simulink model "MODELO_SENOIDAL_SIMPLE"  (R2024b)
settings: Solver=VariableStepAuto  StartTime=0.0  StopTime=10.0  RelTol=1e-3
libraries: simulink x1
settings Model: Creator=RREYM  LastModifiedBy=RREYM

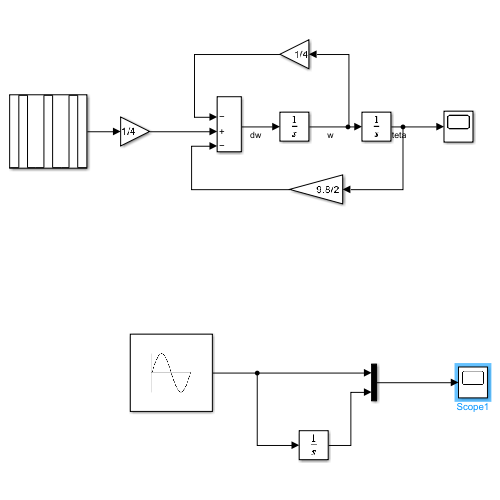
[thumbnail: Simulink's stored preview of the top-level diagram]
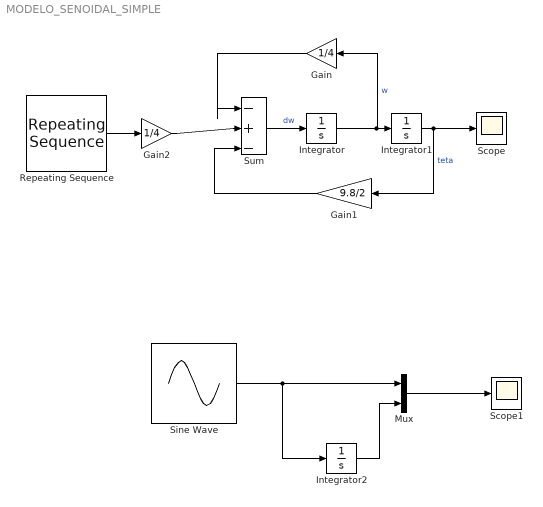
== system MODELO_SENOIDAL_SIMPLE ==
  Gain : Gain  Gain=1/4
  Gain1 : Gain  Gain=9.8/2
  Gain2 : Gain  Gain=1/4
  Integrator : Integrator
  Integrator1 : Integrator
  Integrator2 : Integrator
  Mux : Mux  Inputs=2
  Repeating Sequence : simulink/Sources/Repeating Sequence  rep_seq_t=[0 1 1.001 2 2.001 3]  rep_seq_y=[0 0 1 1 0 0]
  Scope : Scope
  Scope1 : Scope
  Sine Wave : Sin  SampleTime=0
  Sum : Sum  Inputs=|-+-
  wires:
  Repeating Sequence/1 -> Gain2/1
  Gain/1 -> Sum/1
  Sum/1 -> Integrator/1  "dw"
  Gain1/1 -> Sum/3
  Integrator1/1 -> Scope/1, Gain1/1  "teta"
  Integrator/1 -> Gain/1, Integrator1/1  "w"
  Gain2/1 -> Sum/2
  Mux/1 -> Scope1/1
  Integrator2/1 -> Mux/2
  Sine Wave/1 -> Integrator2/1, Mux/1
